simulink model "ABS"  (R2020a)
settings: Solver=FixedStepAuto  StartTime=0.0  StopTime=10  RelTol=1e-3
settings Model: Creator=sadamu  LastModifiedBy=sadamu
settings SolverCC: AutoInsertRateTranBlk=on
settings DataIOCC: LimitDataPoints=on  SaveOutput=off  SignalLogging=off  DSMLogging=off  SaveTime=off
settings OptimizationCC: DefaultParameterBehavior=Inlined  DefaultUnderspecifiedDataType=single  OptimizeBlockIOStorage=off  BufferReuse=off  GlobalBufferReuse=off  ExpressionFolding=off  EnableMemcpy=off  PassReuseOutputArgsThreshold=0  LocalBlockOutputs=off  EfficientFloat2IntCast=on  OptimizeDataStoreBuffers=off  BusAssignmentInplaceUpdate=off  OptimizationLevel=level0  OptimizationPriority=Speed  MultiThreadedLoops=on
settings DebuggingCC: AlgebraicLoopMsg=error  SingleTaskRateTransMsg=error  ParameterTunabilityLossMsg=error  AllowSymbolicDim=off  SFUnexpectedBacktrackingDiag=warning  SFNoUnconditionalDefaultTransitionDiag=warning  SFExecutionAtInitializationDiag=none  ArithmeticOperatorsInVariantConditions=warning
settings SFSimCC: SimUseLocalCustomCode=off  MATLABDynamicMemAlloc=off  CustomCodeUndefinedFunction=UseInterfaceOnly
settings RTWCC: Description=Generic Real-Time Target  GenCodeOnly=on  GenerateReport=on  RTWUseLocalCustomCode=off  BuildConfiguration=Debug  LaunchReport=on
settings CodeAppCC: GenerateComments=off  OperatorAnnotations=on  SimulinkDataObjDesc=on  SFDataObjDesc=on  SimulinkBlockComments=off  EnableCustomComments=on
settings GRTTargetCC: TargetLangStandard=C89/C90 (ANSI)  MatFileLogging=off

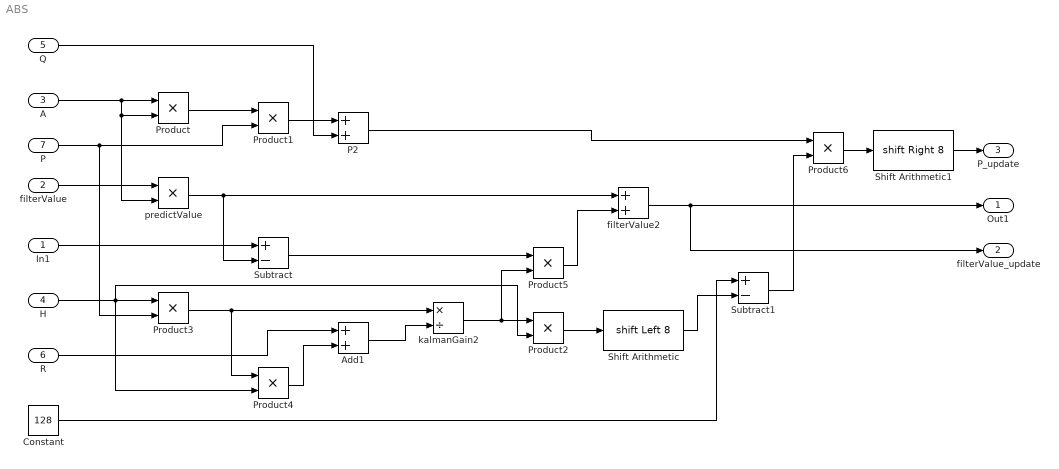
== system ABS ==
  In1 : Inport  OutDataTypeStr=int32  PortDimensions=1
  filterValue : Inport  Port=2  OutDataTypeStr=int32  PortDimensions=1
  A : Inport  Port=3  OutDataTypeStr=int32  PortDimensions=1
  H : Inport  Port=4  OutDataTypeStr=int32  PortDimensions=1
  Q : Inport  Port=5  OutDataTypeStr=int32  PortDimensions=1
  R : Inport  Port=6  OutDataTypeStr=int32  PortDimensions=1
  P : Inport  Port=7  OutDataTypeStr=int32  PortDimensions=1
  Add1 : Sum
  Constant : Constant  Value=128  OutDataTypeStr=int32
  P2 : Sum
  Product{,1..6} (7 alike) : Product  OutDataTypeStr=int32  RndMeth=Simplest
  Shift Arithmetic : ArithShift  BitShiftNumber=8  BitShiftDirection=Left
  Shift Arithmetic1 : ArithShift  BitShiftNumber=8  BitShiftDirection=Right
  Subtract : Sum  Inputs=+-
  Subtract1 : Sum  Inputs=+-
  filterValue2 : Sum
  kalmanGain2 : Product  Inputs=*/  OutDataTypeStr=int32  RndMeth=Simplest
  predictValue : Product  OutDataTypeStr=int32  RndMeth=Simplest
  Out1 : Outport
  filterValue_update : Outport  Port=2
  P_update : Outport  Port=3
  wires:
  Product/1 -> Product1/1
  Product2/1 -> Shift Arithmetic/1
  Product6/1 -> Shift Arithmetic1/1
  Shift Arithmetic1/1 -> P_update/1
  Shift Arithmetic/1 -> Subtract1/2
  Product5/1 -> filterValue2/2
  Subtract1/1 -> Product6/2
  H/1 -> Product2/2, Product3/1, Product4/2
  Subtract/1 -> Product5/1
  Product4/1 -> Add1/2
  In1/1 -> Subtract/1
  Constant/1 -> Subtract1/1
  Add1/1 -> kalmanGain2/2
  P2/1 -> Product6/1
  R/1 -> Add1/1
  Product1/1 -> P2/1
  Q/1 -> P2/2
  filterValue/1 -> predictValue/1
  filterValue2/1 -> Out1/1, filterValue_update/1
  predictValue/1 -> Subtract/2, filterValue2/1
  kalmanGain2/1 -> Product5/2, Product2/1
  Product3/1 -> Product4/1, kalmanGain2/1
  A/1 -> Product/1, predictValue/2, Product/2
  P/1 -> Product3/2, Product1/2
